simulink model "EKF_Harness"  (R2025b)
settings: Solver=FixedStepDiscrete  StartTime=0.0  StopTime=10.0  RelTol=1e-3
Description:
  | Full EKF model harness for IMU/GPS prediction, first-fix LLA-to-NED preprocessing, and StateEstBus verification.
settings Model: DataDictionary=StateEstDict.sldd  Creator=89447  LastModifiedBy=89447

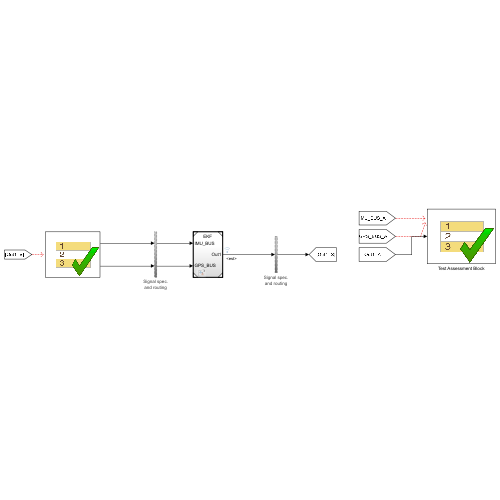
[thumbnail: Simulink's stored preview of the top-level diagram]
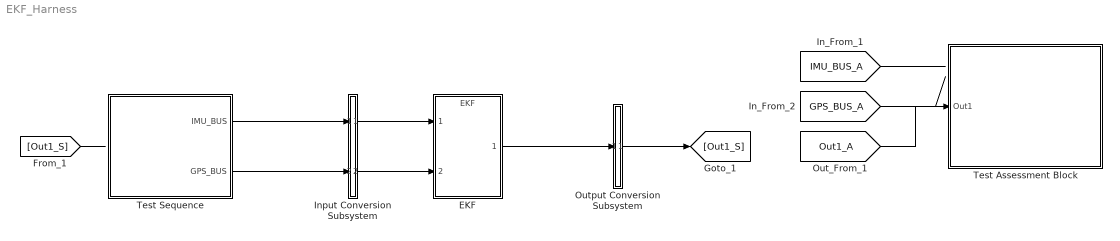
== system EKF_Harness ==
  EKF : ModelReference  ModelNameDialog=EKF  SimulationMode=Normal  ModelReferenceVersion=4.21
  Input Conversion Subsystem : Subsystem  Tag=__SLT_ICS__  Description=|
      | Signal spec.
      | and routing
      settings: AttributesFormatString=%<Description>
  Output Conversion Subsystem : Subsystem  Tag=__SLT_OCS__  Description=|
      | Signal spec.
      | and routing
      settings: AttributesFormatString=%<Description>
  Test Assessment Block : Test Sequence  Tag=__SLT_ASMT__  TreatAsAtomicUnit=on
  Test Sequence : Test Sequence  TreatAsAtomicUnit=on
  wires:
  [IMU_BUS_A] -> ?
  [GPS_BUS_A] -> ?
  [Out1_A] -> Test Assessment Block/1(Out1)
  Test Sequence/1(IMU_BUS) -> Input Conversion Subsystem/1(Inport_1)
  Test Sequence/2(GPS_BUS) -> Input Conversion Subsystem/2(Inport_2)
  [Out1_S] -> ?
  Output Conversion Subsystem/1(Outport_1) -> [Out1_S]
  EKF/1 -> Output Conversion Subsystem/1(Inport_1)
  Input Conversion Subsystem/1(Outport_1) -> EKF/1
  Input Conversion Subsystem/2(Outport_2) -> EKF/2

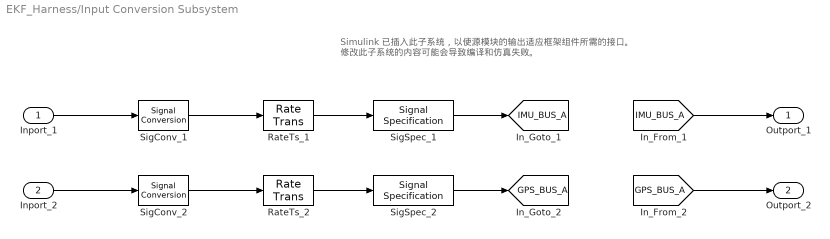
== system EKF_Harness/Input Conversion Subsystem ==
  note: Simulink 已插入此子系统，以使源模块的输出适应框架组件所需的接口。
      |  修改此子系统的内容可能会导致编译和仿真失败。
  Inport_1 : Inport
  Inport_2 : Inport  Port=2
  RateTs_1 : RateTransition  OutPortSampleTime=0.001
  RateTs_2 : RateTransition  OutPortSampleTime=0.001
  SigConv_1 : SignalConversion  ConversionOutput=Virtual bus  OverrideOpt=off
  SigConv_2 : SignalConversion  ConversionOutput=Virtual bus  OverrideOpt=off
  SigSpec_1 : SignalSpecification  OutDataTypeStr=Bus: IMU_BUS  SampleTime=0.001
  SigSpec_2 : SignalSpecification  OutDataTypeStr=Bus: GPS_BUS  SampleTime=0.001
  Outport_1 : Outport
  Outport_2 : Outport  Port=2
  tag scope: GPS_BUS_A=global, IMU_BUS_A=global
  wires:
  [IMU_BUS_A] -> Outport_1/1
  SigSpec_1/1 -> [IMU_BUS_A]
  RateTs_1/1 -> SigSpec_1/1
  SigConv_1/1 -> RateTs_1/1
  Inport_1/1 -> SigConv_1/1
  [GPS_BUS_A] -> Outport_2/1
  SigSpec_2/1 -> [GPS_BUS_A]
  RateTs_2/1 -> SigSpec_2/1
  SigConv_2/1 -> RateTs_2/1
  Inport_2/1 -> SigConv_2/1

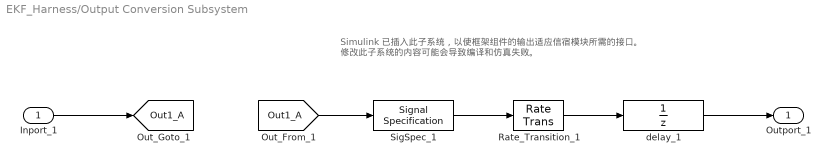
== system EKF_Harness/Output Conversion Subsystem ==
  note: Simulink 已插入此子系统，以使框架组件的输出适应信宿模块所需的接口。
      |  修改此子系统的内容可能会导致编译和仿真失败。
  Inport_1 : Inport
  Rate_Transition_1 : RateTransition  OutPortSampleTimeOpt=Inherit
  SigSpec_1 : SignalSpecification  OutDataTypeStr=Bus: StateEstBus  Dimensions=[1]  SampleTime=0.001
  delay_1 : UnitDelay  SampleTime=-1
  Outport_1 : Outport
  tag scope: Out1_A=global
  wires:
  Inport_1/1 -> [Out1_A]
  [Out1_A] -> SigSpec_1/1
  SigSpec_1/1 -> Rate_Transition_1/1
  Rate_Transition_1/1 -> delay_1/1
  delay_1/1 -> Outport_1/1

== stateflow chart EKF_Harness/Test Assessment Block ==
  state Run
    state step_1_1
      if t > 0.005
      verify(norm(Out1.Position_NED) < 1.0e-6,'EKF_InvalidIMU:PositionHeld','Position must remain at dictionary initial state while IMU is invalid');
      verify(norm(Out1.Velocity_NED) < 1.0e-6,'EKF_InvalidIMU:VelocityHeld','Velocity must remain at dictionary initial state while IMU is invalid');
      verify(abs(norm(Out1.Attitude_quat)-1.0) < 1.0e-6,'EKF_InvalidIMU:QuaternionHeld','Quaternion must remain unit norm while IMU is invalid');
      end
      settings: description=Invalid IMU and GPS must not move the EKF state.
    state step_1_2
      if t > 0.03
      verify(all(isfinite(Out1.Position_NED)),'EKF_FirstFix:PositionFinite','Position must remain finite after first GPS fix');
      verify(norm(Out1.Position_NED) < 0.05,'EKF_FirstFix:OriginNearZero','First GPS fix must define the local NED origin');
      verify(all(isfinite(Out1.Attitude_quat)),'EKF_FirstFix:QuaternionFinite','Quaternion must remain finite');
      verify(abs(norm(Out1.Attitude_quat)-1.0) < 1.0e-3,'EKF_FirstFix:QuaternionUnitNorm','Quaternion norm must remain one');
      end
      settings: description=First valid GPS fix defines local NED origin.
    state step_1_3
      if t > 0.08
      verify(all(isfinite(Out1.Position_NED)),'EKF_NorthMove:PositionFinite','Position must remain finite after northward GPS movement');
      verify(Out1.Position_NED(1) > 0.0,'EKF_NorthMove:NorthPositive','North position estimate must become positive');
      verify(abs(Out1.Position_NED(2)) < 0.5,'EKF_NorthMove:EastNearZero','East position estimate must remain near zero');
      verify(abs(Out1.Position_NED(3)) < 0.5,'EKF_NorthMove:DownNearZero','Down position estimate must remain near zero');
      end
      settings: description=Second GPS fix moves approximately 10 m north.
    state step_1_4
      if t > 0.13
      verify(all(isfinite(Out1.Position_NED)),'EKF_AltitudeMove:PositionFinite','Position must remain finite after altitude change');
      verify(Out1.Position_NED(1) > 0.0,'EKF_AltitudeMove:NorthRemainsPositive','North estimate must retain northward displacement');
      verify(Out1.Position_NED(3) < 0.0,'EKF_AltitudeMove:DownNegative','Higher GPS altitude must map to negative NED Down');
      end
      settings: description=Third GPS fix increases altitude by 5 m.
    (default) -> (junction 22)
    Run -> (junction 22)
    (junction 22) -> (junction 23) [order 1] : [t < 0.02
        | ]
    (junction 23) -> step_1_1 [order 1] : [~in(Run.step_1_1)]
    (junction 22) -> (junction 31) [order 2]
    (junction 23) -> (junction 26) [order 2]
    (junction 31) -> (junction 32) [order 1] : [t < 0.07
        | ]
    (junction 32) -> step_1_2 [order 1] : [~in(Run.step_1_2)]
    (junction 31) -> (junction 46) [order 2]
    (junction 32) -> (junction 35) [order 2]
    (junction 46) -> (junction 47) [order 1] : [t < 0.12
        | ]
    (junction 47) -> step_1_3 [order 1] : [~in(Run.step_1_3)]
    (junction 46) -> (junction 54) [order 2]
    (junction 47) -> (junction 50) [order 2]
    (junction 54) -> (junction 55)
    (junction 55) -> step_1_4 [order 1] : [~in(Run.step_1_4)]
    (junction 55) -> (junction 58) [order 2]
  (default) -> Run
  data: Out1 input Bus: StateEstBus size=[1]

== stateflow chart EKF_Harness/Test Sequence ==
  state Run
    IMU_BUS.Gyro = single([0;0;0]);
    IMU_BUS.Timestamp = t;
    GPS_BUS.Lon = single(-122.140165);
    GPS_BUS.Velocity = single([0;0;0]);
    if t < 0.02
    IMU_BUS.Accel = single([0;0;0]);
    IMU_BUS.Valid = false;
    GPS_BUS.Lat = single(47.641468);
    GPS_BUS.Alt = single(122.0);
    GPS_BUS.Valid = false;
    GPS_BUS.Timestamp = 0.0;
    elseif t < 0.07
    IMU_BUS.Accel = single([0;0;-9.81]);
    IMU_BUS.Valid = true;
    GPS_BUS.Lat = single(47.641468);
    GPS_BUS.Alt = single(122.0);
    GPS_BUS.Valid = true;
    GPS_BUS.Timestamp = 1.0;
    elseif t < 0.12
    IMU_BUS.Accel = single([0;0;-9.81]);
    IMU_BUS.Valid = true;
    GPS_BUS.Lat = single(47.641468 + 10.0/6378137.0*180.0/pi);
    GPS_BUS.Alt = single(122.0);
    GPS_BUS.Valid = true;
    GPS_BUS.Timestamp = 2.0;
    else
    IMU_BUS.Accel = single([0;0;-9.81]);
    IMU_BUS.Valid = true;
    GPS_BUS.Lat = single(47.641468 + 10.0/6378137.0*180.0/pi);
    GPS_BUS.Alt = single(127.0);
    GPS_BUS.Valid = true;
    GPS_BUS.Timestamp = 3.0;
    end
    settings: description=Invalid sensor startup, first GPS origin, 10 m north movement, then 5 m altitude increase.
  (default) -> Run
  data: IMU_BUS output Bus: IMU_BUS size=[1]; GPS_BUS output Bus: GPS_BUS size=[1]
